simulink model "esempioS"  (R2021a)
settings: Solver=VariableStepAuto  StartTime=0.0  StopTime=10.0  RelTol=1e-3
values from neighbouring files (symbols this model uses):
  Ahat = A-B*K    [esempio.m]    (also in esempio1.m; esempio2.m)
  B = [ 0; 1]    [esempio.m]    (also in esempio1.m = [0; 1]; esempio2.m = [0; 1])
  C = eye(2)    [esempio.m]    (also in esempio1.m; esempio2.m)
  D = zeros(2,1)    [esempio.m]    (also in esempio1.m; esempio2.m)
settings Model: Creator=itama  LastModifiedBy=itama
settings SolverCC: AlgebraicLoopSolver=TrustRegion
settings DebuggingCC: SFMachineParentedDataDiag=warning

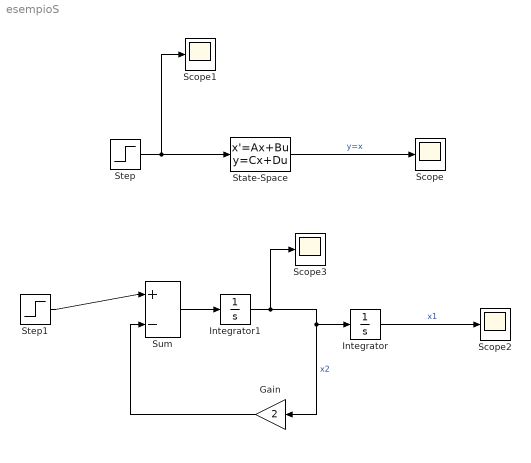
== system esempioS ==
  Gain : Gain  Gain=2
  Integrator : Integrator
  Integrator1 : Integrator
  Scope{,1..3} (4 alike) : Scope
  State-Space : StateSpace  A=Ahat  B=B  C=C  D=D  InitialCondition=[0;0]
  Step : Step  SampleTime=0
  Step1 : Step  SampleTime=0
  Sum : Sum  Inputs=|+-
  wires:
  State-Space/1 -> Scope/1  "y=x"
  Step/1 -> State-Space/1, Scope1/1
  Integrator/1 -> Scope2/1  "x1"
  Integrator1/1 -> Scope3/1, Gain/1, Integrator/1  "x2"
  Sum/1 -> Integrator1/1
  Gain/1 -> Sum/2
  Step1/1 -> Sum/1
